simulink model "MODBUS_v2018"  (R2018a)
settings: Solver=FixedStepDiscrete  StartTime=0.0  StopTime=inf  FixedStep=1  MaxStep=0.2  RelTol=1e-3
libraries: modbusMatLib x2, realtime_pacer_lib x1
settings Model: Creator=jvl  LastModifiedBy=jvl

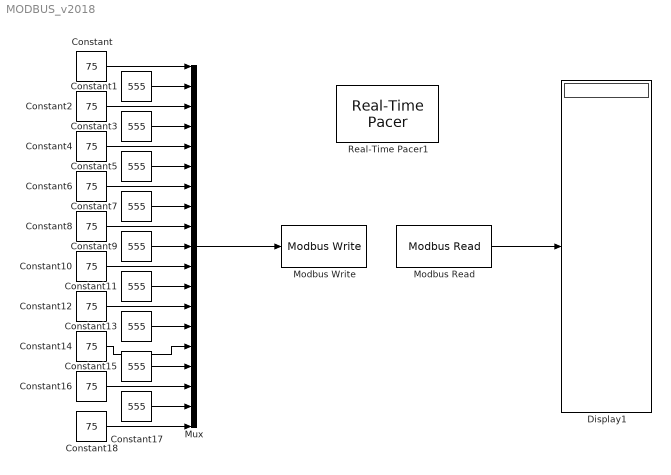
== system MODBUS_v2018 ==
  Constant{,2,4,6,8,10,12,14,16,18} (10 alike) : Constant  Value=75
  Constant{1,3,5,7,9,11,13,15,17} (9 alike) : Constant  Value=555
  Display1 : Display
  Modbus Read : modbusMatLib/Modbus Read  registry=001  ipAddress='192.168.100.40'  port=502
  Modbus Write : modbusMatLib/Modbus Write  registry=001  port=502  ipAddress='192.168.100.40'
  Mux : Mux  Inputs=19
  Real-Time Pacer1 : realtime_pacer_lib/Real-Time Pacer  simTimePerRealTime=1
  wires:
  Constant/1 -> Mux/1
  Modbus Read/1 -> Display1/1
  Mux/1 -> Modbus Write/1
  Constant1/1 -> Mux/2
  Constant2/1 -> Mux/3
  Constant4/1 -> Mux/5
  Constant6/1 -> Mux/7
  Constant8/1 -> Mux/9
  Constant10/1 -> Mux/11
  Constant12/1 -> Mux/13
  Constant14/1 -> Mux/15
  Constant3/1 -> Mux/4
  Constant5/1 -> Mux/6
  Constant7/1 -> Mux/8
  Constant9/1 -> Mux/10
  Constant11/1 -> Mux/12
  Constant13/1 -> Mux/14
  Constant15/1 -> Mux/16
  Constant16/1 -> Mux/17
  Constant17/1 -> Mux/18
  Constant18/1 -> Mux/19
